simulink subsystem "Baseline"  (R2024a)
settings: Solver=VariableStepAuto  StartTime=0.0  StopTime=10.0  RelTol=1e-3
undefined symbols (not defined in the file): Baseline, ControllersLib, SimIn, SimPar
libraries: ComponentsLib x12, AdaptiveLib x1, libAxisTransformations x1
settings Model: Creator=tbritton  LastModifiedBy=azmol
settings SolverCC: AlgebraicLoopSolver=TrustRegion
settings OptimizationCC: ReuseModelBlockBuffer=off
settings DebuggingCC: UnconnectedInputMsg=warning  UnconnectedOutputMsg=warning  UnconnectedLineMsg=warning
settings ModelReferenceCC: EnableRefExpFcnMdlSchedulingChecks=on
settings RTWCC: GPUComputeCapability=3.5  DLArmComputeVersion=19.05

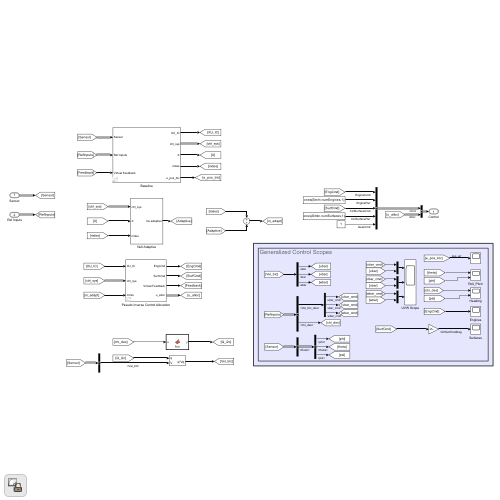
[thumbnail: Simulink's stored preview of the top-level diagram]
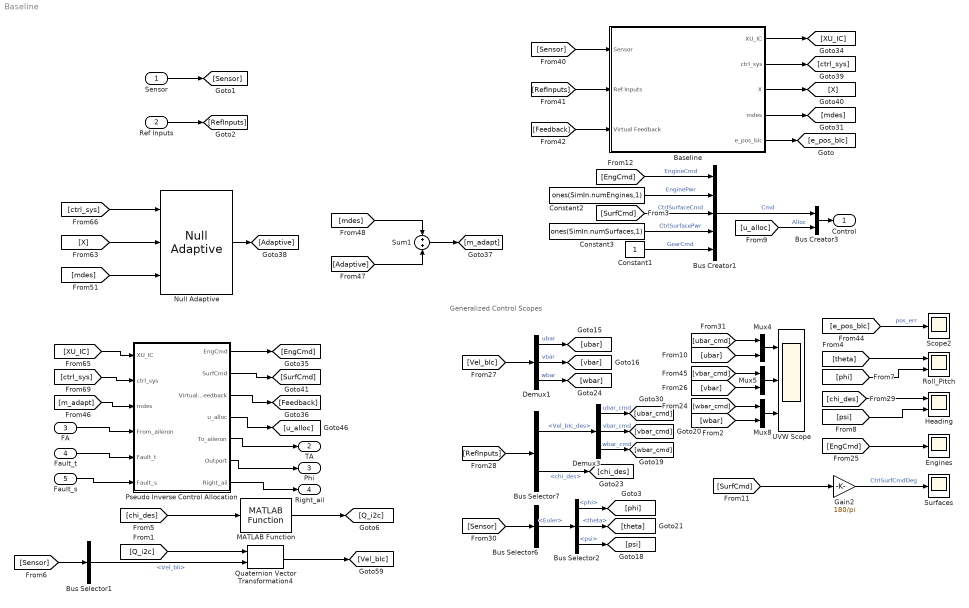
== system Baseline ==
  note: Generalized Control Scopes
  Sensor : Inport  OutDataTypeStr=Bus: SensorBus
  Ref Inputs : Inport  Port=2  OutDataTypeStr=Bus: BUS_REF_INPUT
  FA : Inport  Port=3
  Fault_t : Inport  Port=4
  Fault_s : Inport  Port=5
  Baseline : Subsystem  AncestorBlock=ControllersLib/Baseline
      settings: LibrarySourceBlock=ControllersLib/Baseline
  Bus Creator1 : BusCreator  Inputs=5  OutDataTypeStr=Bus: BUS_CMD
  Bus Creator3 : BusCreator  Inputs=2
  Bus Selector1 : BusSelector  OutputSignals=Vel_bIi
  Bus Selector2 : BusSelector  OutputSignals=phi,theta,psi
  Bus Selector6 : BusSelector  OutputSignals=Euler
  Bus Selector7 : BusSelector  OutputSignals=Vel_bIc_des,chi_des
  Constant1 : Constant
  Constant2 : Constant  Value=ones(SimIn.numEngines,1)
  Constant3 : Constant  Value=ones(SimIn.numSurfaces,1)
  Demux1 : Demux  Outputs=3
  Demux3 : Demux  Outputs=3
  Engines : Scope
  Gain2 : Gain  Gain=180/pi
  Heading : Scope  NumInputPorts=2
  MATLAB Function : ComponentsLib/ConvertToControlFrame/MATLAB Function  SystemSampleTime=-1  VariantActivationTime=update diagram  AllowFlexibleInterface=on  Latency=0  AutoFrameSizeCalculation=off
      settings: SourceProductName=Components
  Mux4 : Mux  Inputs=2
  Mux5 : Mux  Inputs=2
  Mux8 : Mux  Inputs=2
  Null Adaptive : AdaptiveLib/Null Adaptive  SystemSampleTime=-1  VariantActivationTime=update diagram  AllowFlexibleInterface=on  Latency=0  AutoFrameSizeCalculation=off
      settings: SourceProductName=Adaptive Augmentation
  Pseudo Inverse Control Allocation : Subsystem  AncestorBlock=AllocatorsLib/Pseudo Inverse Control Allocation
      settings: LibrarySourceBlock=AllocatorsLib/Pseudo Inverse Control Allocation
  Quaternion Vector Transformation4 : libAxisTransformations/Quaternion Vector Transformation  n=0
  Roll_Pitch : Scope  NumInputPorts=2
  Scope2 : Scope
  Sum1 : Sum
  Surfaces : Scope
  UVW Scope : Scope  NumInputPorts=3
  Control : Outport  OutDataTypeStr=Bus: BUS_CONTROL  VectorParamsAs1DForOutWhenUnconnected=off
  TA : Outport  Port=2
  Phi : Outport  Port=3
  Right_ail : Outport  Port=4
  wires:
  Baseline/5(e_pos_blc) -> [e_pos_bIc]
  Demux1/1 -> [ubar]  "ubar"
  Mux4/1 -> UVW Scope/1
  Demux3/3 -> [wbar_cmd]  "wbar_cmd"
  Mux5/1 -> UVW Scope/2
  [vbar_cmd] -> Mux5/1
  [ubar_cmd] -> Mux4/1
  [vbar] -> Mux5/2
  [SurfCmd] -> Gain2/1
  [chi_des] -> Heading/1
  [ubar] -> Mux4/2
  [Sensor] -> Bus Selector6/1
  [RefInputs] -> Bus Selector7/1
  [wbar] -> Mux8/2
  [phi] -> Roll_Pitch/2
  Demux3/2 -> [vbar_cmd]  "vbar_cmd"
  [e_pos_bIc] -> Scope2/1  "pos_err"
  Bus Selector6/1 -> Bus Selector2/1  "<Euler>"
  Bus Selector2/1 -> [phi]  "<phi>"
  Mux8/1 -> UVW Scope/3
  Bus Selector2/3 -> [psi]  "<psi>"
  Gain2/1 -> Surfaces/1  "CtrlSurfCmdDeg"
  [theta] -> Roll_Pitch/1
  Bus Selector2/2 -> [theta]  "<theta>"
  [psi] -> Heading/2
  Demux1/2 -> [vbar]  "vbar"
  [EngCmd] -> Engines/1
  Bus Selector7/1 -> Demux3/1  "<Vel_bIc_des>"
  Demux3/1 -> [ubar_cmd]  "ubar_cmd"
  [Vel_bIc] -> Demux1/1
  Bus Selector7/2 -> [chi_des]  "<chi_des>"
  [wbar_cmd] -> Mux8/1
  Demux1/3 -> [wbar]  "wbar"
  [Sensor] -> Bus Selector1/1
  MATLAB Function/1 -> [Q_i2c]
  Quaternion Vector Transformation4/1 -> [Vel_bIc]
  [chi_des] -> MATLAB Function/1
  [Q_i2c] -> Quaternion Vector Transformation4/1
  Bus Selector1/1 -> Quaternion Vector Transformation4/2  "<Vel_bIi>"
  [ctrl_sys] -> Pseudo Inverse Control Allocation/2(ctrl_sys)
  [XU_IC] -> Pseudo Inverse Control Allocation/1(XU_IC)
  Pseudo Inverse Control Allocation/4(u_alloc) -> [u_alloc]
  Pseudo Inverse Control Allocation/2(SurfCmd) -> [SurfCmd]
  [Adaptive] -> Sum1/2
  [mdes] -> Sum1/1
  Sum1/1 -> [m_adapt]
  Baseline/3(X) -> [X]
  Baseline/2(ctrl_sys) -> [ctrl_sys]
  Null Adaptive/1 -> [Adaptive]
  [X] -> Null Adaptive/2
  [mdes] -> Null Adaptive/3
  [ctrl_sys] -> Null Adaptive/1
  Pseudo Inverse Control Allocation/1(EngCmd) -> [EngCmd]
  Baseline/1(XU_IC) -> [XU_IC]
  Pseudo Inverse Control Allocation/3(Virtual Feedback) -> [Feedback]
  [m_adapt] -> Pseudo Inverse Control Allocation/3(mdes)
  Baseline/4(mdes) -> [mdes]
  [Feedback] -> Baseline/3(Virtual Feedback)
  [RefInputs] -> Baseline/2(Ref Inputs)
  [Sensor] -> Baseline/1(Sensor)
  Constant3/1 -> Bus Creator1/4  "CtrlSurfacePwr"
  Constant2/1 -> Bus Creator1/2  "EnginePwr"
  [EngCmd] -> Bus Creator1/1  "EngineCmd"
  Sensor/1 -> [Sensor]
  Bus Creator1/1 -> Bus Creator3/1  "Cmd"
  [SurfCmd] -> Bus Creator1/3  "CtrlSurfaceCmd"
  Constant1/1 -> Bus Creator1/5  "GearCmd"
  Bus Creator3/1 -> Control/1
  [u_alloc] -> Bus Creator3/2  "Alloc"
  Ref Inputs/1 -> [RefInputs]
  FA/1 -> Pseudo Inverse Control Allocation/4(From_aileron)
  Pseudo Inverse Control Allocation/5(To_aileron) -> TA/1
  Pseudo Inverse Control Allocation/6(Outport) -> Phi/1
  Fault_t/1 -> Pseudo Inverse Control Allocation/5(Fault_t)
  Fault_s/1 -> Pseudo Inverse Control Allocation/6(Fault_s)
  Pseudo Inverse Control Allocation/7(Right_ail) -> Right_ail/1

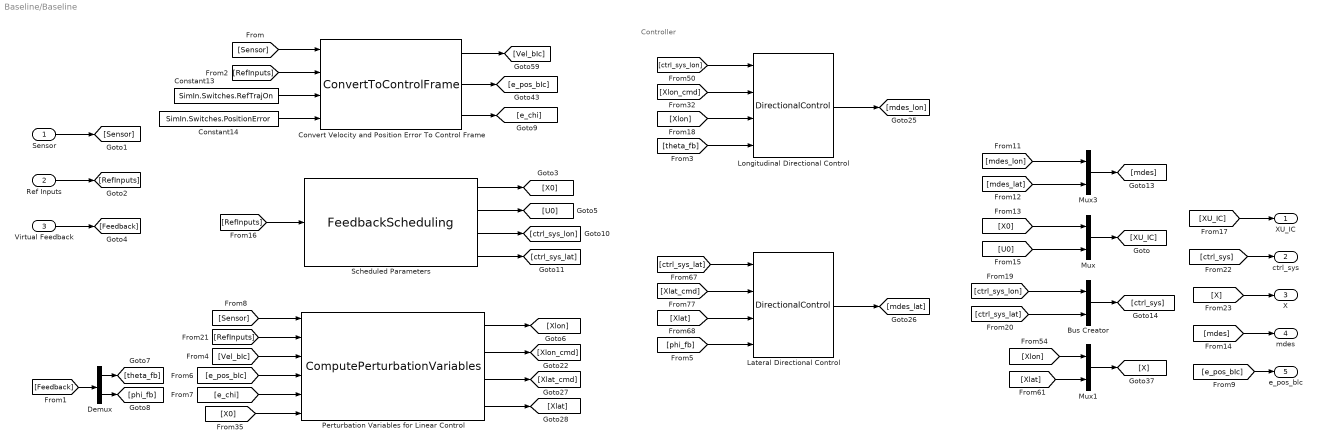
== system Baseline/Baseline ==
  note: Controller
  Sensor : Inport  OutDataTypeStr=Bus: SensorBus
  Ref Inputs : Inport  Port=2  OutDataTypeStr=Bus: BUS_REF_INPUT
  Virtual Feedback : Inport  Port=3
  Bus Creator : BusCreator  Inputs=2
  Constant13 : Constant  Value=SimIn.Switches.RefTrajOn
  Constant14 : Constant  Value=SimIn.Switches.PositionError
  Convert Velocity and Position Error To Control Frame : ComponentsLib/ConvertToControlFrame  SystemSampleTime=-1  VariantActivationTime=update diagram  AllowFlexibleInterface=on  Latency=0  AutoFrameSizeCalculation=off
      settings: SourceProductName=Components
  Demux : Demux  Outputs=2
  Lateral Directional Control : ComponentsLib/DirectionalControl  SystemSampleTime=-1  VariantActivationTime=update diagram  AllowFlexibleInterface=on  Latency=0  AutoFrameSizeCalculation=off
      settings: SourceProductName=Components
  Longitudinal Directional Control : ComponentsLib/DirectionalControl  SystemSampleTime=-1  VariantActivationTime=update diagram  AllowFlexibleInterface=on  Latency=0  AutoFrameSizeCalculation=off
      settings: SourceProductName=Components
  Mux : Mux  Inputs=2
  Mux1 : Mux  Inputs=2
  Mux3 : Mux  Inputs=2
  Perturbation Variables for Linear Control : ComponentsLib/ComputePerturbationVariables  SystemSampleTime=-1  VariantActivationTime=update diagram  AllowFlexibleInterface=on  Latency=0  AutoFrameSizeCalculation=off
      settings: SourceProductName=Components
  Scheduled Parameters : ComponentsLib/FeedbackScheduling  SystemSampleTime=-1  VariantActivationTime=update diagram  AllowFlexibleInterface=on  Latency=0  AutoFrameSizeCalculation=off
      settings: SourceProductName=Components
  XU_IC : Outport
  ctrl_sys : Outport  Port=2
  X : Outport  Port=3
  mdes : Outport  Port=4
  e_pos_blc : Outport  Port=5
  wires:
  [X] -> X/1
  [Xlat] -> Mux1/2
  [Xlon] -> Mux1/1
  Mux1/1 -> [X]
  [ctrl_sys] -> ctrl_sys/1
  Bus Creator/1 -> [ctrl_sys]
  [ctrl_sys_lat] -> Bus Creator/2
  [ctrl_sys_lon] -> Bus Creator/1
  [XU_IC] -> XU_IC/1
  Mux/1 -> [XU_IC]
  [U0] -> Mux/2
  [X0] -> Mux/1
  [mdes] -> mdes/1
  Mux3/1 -> [mdes]
  [mdes_lat] -> Mux3/2
  [mdes_lon] -> Mux3/1
  [phi_fb] -> Lateral Directional Control/4
  [theta_fb] -> Longitudinal Directional Control/4
  Demux/1 -> [theta_fb]
  Demux/2 -> [phi_fb]
  [Feedback] -> Demux/1
  Virtual Feedback/1 -> [Feedback]
  [Xlat_cmd] -> Lateral Directional Control/2
  [Xlon] -> Longitudinal Directional Control/3
  [Xlat] -> Lateral Directional Control/3
  Longitudinal Directional Control/1 -> [mdes_lon]
  [ctrl_sys_lon] -> Longitudinal Directional Control/1
  [ctrl_sys_lat] -> Lateral Directional Control/1
  Lateral Directional Control/1 -> [mdes_lat]
  [Xlon_cmd] -> Longitudinal Directional Control/2
  Scheduled Parameters/4 -> [ctrl_sys_lat]
  Scheduled Parameters/2 -> [U0]
  [e_chi] -> Perturbation Variables for Linear Control/5
  Constant14/1 -> Convert Velocity and Position Error To Control Frame/4
  [RefInputs] -> Perturbation Variables for Linear Control/2
  Constant13/1 -> Convert Velocity and Position Error To Control Frame/3
  [Vel_bIc] -> Perturbation Variables for Linear Control/3
  [Sensor] -> Convert Velocity and Position Error To Control Frame/1
  Convert Velocity and Position Error To Control Frame/3 -> [e_chi]
  Perturbation Variables for Linear Control/2 -> [Xlon_cmd]
  [RefInputs] -> Scheduled Parameters/1
  Perturbation Variables for Linear Control/4 -> [Xlat]
  [e_pos_bIc] -> Perturbation Variables for Linear Control/4
  Scheduled Parameters/3 -> [ctrl_sys_lon]
  Convert Velocity and Position Error To Control Frame/2 -> [e_pos_bIc]
  Convert Velocity and Position Error To Control Frame/1 -> [Vel_bIc]
  [RefInputs] -> Convert Velocity and Position Error To Control Frame/2
  Ref Inputs/1 -> [RefInputs]
  Scheduled Parameters/1 -> [X0]
  Sensor/1 -> [Sensor]
  Perturbation Variables for Linear Control/3 -> [Xlat_cmd]
  [Sensor] -> Perturbation Variables for Linear Control/1
  Perturbation Variables for Linear Control/1 -> [Xlon]
  [X0] -> Perturbation Variables for Linear Control/6
  [e_pos_bIc] -> e_pos_blc/1

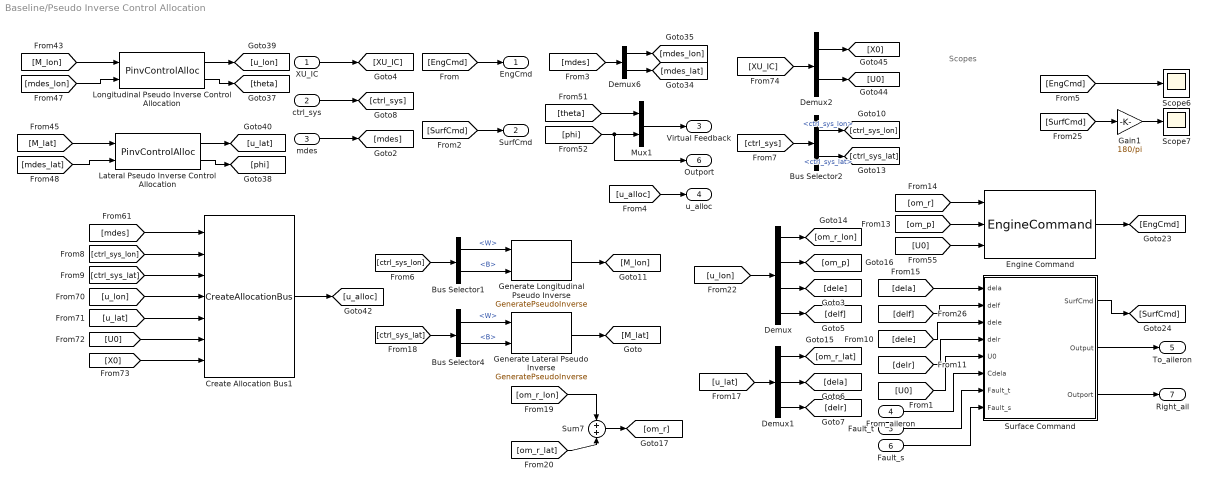
== system Baseline/Pseudo Inverse Control Allocation ==
  note: Scopes
  XU_IC : Inport
  ctrl_sys : Inport  Port=2
  mdes : Inport  Port=3
  From_aileron : Inport  Port=4
  Fault_t : Inport  Port=5
  Fault_s : Inport  Port=6
  Bus Selector1 : BusSelector  OutputSignals=W,B
  Bus Selector2 : BusSelector  OutputSignals=ctrl_sys_lon,ctrl_sys_lat
  Bus Selector4 : BusSelector  OutputSignals=W,B
  Create Allocation Bus1 : ComponentsLib/CreateAllocationBus  SystemSampleTime=-1  VariantActivationTime=update diagram  AllowFlexibleInterface=on  Latency=0  AutoFrameSizeCalculation=off
      settings: SourceProductName=Components
  Demux : Demux  Outputs=[8 1 1 1]
  Demux1 : Demux  Outputs=[8 1 1]
  Demux2 : Demux  Outputs=[12 13]
  Demux6 : Demux  Outputs=[3 3]
  Engine Command : ComponentsLib/EngineCommand  SystemSampleTime=-1  VariantActivationTime=update diagram  AllowFlexibleInterface=on  Latency=0  AutoFrameSizeCalculation=off
      settings: SourceProductName=Components
  Gain1 : Gain  Gain=180/pi
  Generate Lateral Pseudo Inverse : ComponentsLib/GeneratePseudoInverse  SystemSampleTime=-1  VariantActivationTime=update diagram  AllowFlexibleInterface=on  Latency=0  AutoFrameSizeCalculation=off
      settings: SourceProductName=Components
  Generate Longitudinal Pseudo Inverse : ComponentsLib/GeneratePseudoInverse  SystemSampleTime=-1  VariantActivationTime=update diagram  AllowFlexibleInterface=on  Latency=0  AutoFrameSizeCalculation=off
      settings: SourceProductName=Components
  Lateral Pseudo Inverse Control Allocation : ComponentsLib/PinvControlAlloc  SystemSampleTime=-1  VariantActivationTime=update diagram  AllowFlexibleInterface=on  Latency=0  AutoFrameSizeCalculation=off
      settings: SourceProductName=Components
  Longitudinal Pseudo Inverse Control Allocation : ComponentsLib/PinvControlAlloc  SystemSampleTime=-1  VariantActivationTime=update diagram  AllowFlexibleInterface=on  Latency=0  AutoFrameSizeCalculation=off
      settings: SourceProductName=Components
  Mux1 : Mux  Inputs=2
  Scope6 : Scope
  Scope7 : Scope
  Sum7 : Sum
  Surface Command : Subsystem  AncestorBlock=ComponentsLib/SurfaceCommand
  EngCmd : Outport
  SurfCmd : Outport  Port=2
  Virtual Feedback : Outport  Port=3
  u_alloc : Outport  Port=4
  To_aileron : Outport  Port=5
  Outport : Outport  Port=6
  Right_ail : Outport  Port=7
  wires:
  Surface Command/3(Outport) -> Right_ail/1
  Fault_s/1 -> Surface Command/8(Fault_s)
  Fault_t/1 -> Surface Command/7(Fault_t)
  From_aileron/1 -> Surface Command/6(Cdela)
  Surface Command/2(Output) -> To_aileron/1
  [ctrl_sys_lat] -> Create Allocation Bus1/3
  [ctrl_sys_lon] -> Create Allocation Bus1/2
  Bus Selector2/2 -> [ctrl_sys_lat]  "<ctrl_sys_lat>"
  Bus Selector2/1 -> [ctrl_sys_lon]  "<ctrl_sys_lon>"
  [ctrl_sys] -> Bus Selector2/1
  Bus Selector1/2 -> Generate Longitudinal Pseudo Inverse/2  "<B>"
  Bus Selector4/2 -> Generate Lateral Pseudo Inverse/2  "<B>"
  Generate Lateral Pseudo Inverse/1 -> [M_lat]
  Bus Selector4/1 -> Generate Lateral Pseudo Inverse/1  "<W>"
  Generate Longitudinal Pseudo Inverse/1 -> [M_lon]
  [ctrl_sys_lon] -> Bus Selector1/1
  Bus Selector1/1 -> Generate Longitudinal Pseudo Inverse/1  "<W>"
  [ctrl_sys_lat] -> Bus Selector4/1
  [EngCmd] -> Scope6/1
  [SurfCmd] -> Gain1/1
  Gain1/1 -> Scope7/1
  [u_alloc] -> u_alloc/1
  ctrl_sys/1 -> [ctrl_sys]
  XU_IC/1 -> [XU_IC]
  mdes/1 -> [mdes]
  [mdes] -> Demux6/1
  Demux6/1 -> [mdes_lon]
  Demux6/2 -> [mdes_lat]
  [mdes] -> Create Allocation Bus1/1
  Demux2/1 -> [X0]
  [X0] -> Create Allocation Bus1/7
  [XU_IC] -> Demux2/1
  [u_lat] -> Create Allocation Bus1/5
  Create Allocation Bus1/1 -> [u_alloc]
  [u_lon] -> Create Allocation Bus1/4
  [U0] -> Create Allocation Bus1/6
  Demux2/2 -> [U0]
  [SurfCmd] -> SurfCmd/1
  [EngCmd] -> EngCmd/1
  [dela] -> Surface Command/1(dela)
  [U0] -> Surface Command/5(U0)
  [om_r] -> Engine Command/1
  [om_p] -> Engine Command/2
  [delr] -> Surface Command/4(delr)
  [delf] -> Surface Command/2(delf)
  [dele] -> Surface Command/3(dele)
  [U0] -> Engine Command/3
  Surface Command/1(SurfCmd) -> [SurfCmd]
  Engine Command/1 -> [EngCmd]
  Demux1/3 -> [delr]
  Demux/4 -> [delf]
  Demux/1 -> [om_r_lon]
  Demux1/1 -> [om_r_lat]
  Demux1/2 -> [dela]
  [u_lon] -> Demux/1
  Sum7/1 -> [om_r]
  [om_r_lon] -> Sum7/1
  [om_r_lat] -> Sum7/2
  [u_lat] -> Demux1/1
  Demux/2 -> [om_p]
  Demux/3 -> [dele]
  [M_lat] -> Lateral Pseudo Inverse Control Allocation/1
  [M_lon] -> Longitudinal Pseudo Inverse Control Allocation/1
  Mux1/1 -> Virtual Feedback/1
  Longitudinal Pseudo Inverse Control Allocation/2 -> [theta]
  Lateral Pseudo Inverse Control Allocation/1 -> [u_lat]
  [mdes_lon] -> Longitudinal Pseudo Inverse Control Allocation/2
  [phi] -> Mux1/2, Outport/1
  [mdes_lat] -> Lateral Pseudo Inverse Control Allocation/2
  [theta] -> Mux1/1
  Longitudinal Pseudo Inverse Control Allocation/1 -> [u_lon]
  Lateral Pseudo Inverse Control Allocation/2 -> [phi]

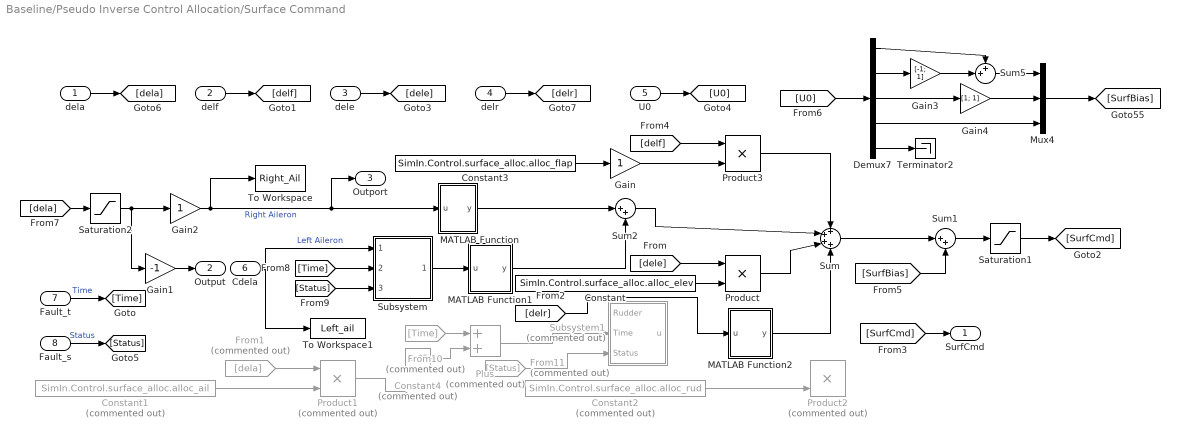
== system Baseline/Pseudo Inverse Control Allocation/Surface Command ==
  dela : Inport
  delf : Inport  Port=2
  dele : Inport  Port=3
  delr : Inport  Port=4
  U0 : Inport  Port=5
  Cdela : Inport  Port=6
  Fault_t : Inport  Port=7
  Fault_s : Inport  Port=8
  Constant : Constant  Value=SimIn.Control.surface_alloc.alloc_elev
  Constant1 : Constant  Commented=on  Value=SimIn.Control.surface_alloc.alloc_ail
  Constant2 : Constant  Commented=on  Value=SimIn.Control.surface_alloc.alloc_rud
  Constant3 : Constant  Value=SimIn.Control.surface_alloc.alloc_flap
  Constant4 : Constant  Commented=on  Value=-0.05
  Demux7 : Demux  Outputs=[1 1 1 1 -1]
  From1 : From  Commented=on  GotoTag=dela
  From10 : From  Commented=on  GotoTag=Time
  From11 : From  Commented=on  GotoTag=Status
  Gain : Gain
  Gain1 : Gain  Gain=-1
  Gain2 : Gain
  Gain3 : Gain  Gain=[-1; 1]
  Gain4 : Gain  Gain=[1; 1]
  MATLAB Function : MATLAB Function  TreatAsAtomicUnit=on
  MATLAB Function1 : MATLAB Function  TreatAsAtomicUnit=on
  MATLAB Function2 : MATLAB Function  TreatAsAtomicUnit=on
  Mux4 : Mux  Inputs=3
  Plus : Sum  Commented=on
  Product : Product
  Product1 : Product  Commented=on
  Product2 : Product  Commented=on
  Product3 : Product
  Saturation1 : Saturate  UpperLimit=SimPar.Actuator.MaxPos  LowerLimit=SimPar.Actuator.MinPos
  Saturation2 : Saturate  UpperLimit=0.44  LowerLimit=-0.44
  Subsystem : Subsystem
  Subsystem1 : Subsystem  Commented=on
  Sum : Sum  Inputs=++++
  Sum1 : Sum  Inputs=|++
  Sum2 : Sum  Inputs=|++
  Sum5 : Sum  Inputs=++|
  Terminator2 : Terminator
  To Workspace : ToWorkspace  VariableName=Right_Ail  SaveFormat=Timeseries  SampleTime=-1
  To Workspace1 : ToWorkspace  VariableName=Left_ail  SaveFormat=Timeseries  SampleTime=-1
  SurfCmd : Outport
  Output : Outport  Port=2
  Outport : Outport  Port=3
  wires:
  [delr] -> MATLAB Function2/1(u)
  From11/1 -> Subsystem1/3(Status)
  Plus/1 -> Subsystem1/2(Time)
  [Status] -> Subsystem/3(Inport1)
  [Time] -> Subsystem/2(Inport)
  Fault_s/1 -> [Status]  "Status"
  Fault_t/1 -> [Time]  "Time"
  Constant2/1 -> Product2/2
  Subsystem/1(Out1) -> MATLAB Function1/1(u)
  Cdela/1 -> Subsystem/1(Left Aileron), To Workspace1/1  "Left Aileron"
  Saturation2/1 -> Gain1/1, Gain2/1
  MATLAB Function1/1(y) -> Sum2/2
  MATLAB Function/1(y) -> Sum2/1
  Gain1/1 -> Output/1
  Gain2/1 -> To Workspace/1, MATLAB Function/1(u), Outport/1  "Right Aileron"
  [dela] -> Saturation2/1
  Gain/1 -> Product3/2
  [delf] -> Product3/1
  Constant3/1 -> Gain/1
  Product3/1 -> Sum/1
  [SurfBias] -> Sum1/2
  Sum/1 -> Sum1/1
  Sum1/1 -> Saturation1/1
  MATLAB Function2/1(y) -> Sum/4
  Product/1 -> Sum/3
  Constant/1 -> Product/2
  [dele] -> Product/1
  U0/1 -> [U0]
  Gain4/1 -> Mux4/2
  Demux7/1 -> Sum5/1
  Demux7/5 -> Terminator2/1
  Gain3/1 -> Sum5/2
  Demux7/3 -> Gain4/1
  Demux7/4 -> Mux4/3
  [U0] -> Demux7/1
  Mux4/1 -> [SurfBias]
  Demux7/2 -> Gain3/1
  Sum5/1 -> Mux4/1
  Saturation1/1 -> [SurfCmd]
  [SurfCmd] -> SurfCmd/1
  delf/1 -> [delf]
  delr/1 -> [delr]
  dela/1 -> [dela]
  dele/1 -> [dele]
  From1/1 -> Product1/1
  Constant1/1 -> Product1/2
  Product1/1 -> ?
  Sum2/1 -> Sum/2
  From10/1 -> Plus/1
  Constant4/1 -> Plus/2

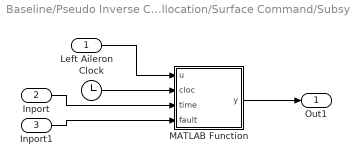
== system Baseline/Pseudo Inverse Control Allocation/Surface Command/Subsystem ==
  Left Aileron : Inport
  Inport : Inport  Port=2
  Inport1 : Inport  Port=3
  Clock : Clock
  MATLAB Function : MATLAB Function  TreatAsAtomicUnit=on
  Out1 : Outport
  wires:
  Inport1/1 -> MATLAB Function/4(fault)
  Inport/1 -> MATLAB Function/3(time)
  MATLAB Function/1(y) -> Out1/1
  Left Aileron/1 -> MATLAB Function/1(u)
  Clock/1 -> MATLAB Function/2(cloc)

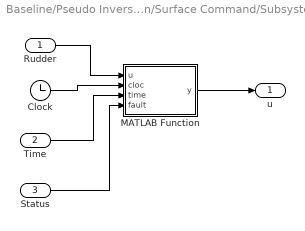
== system Baseline/Pseudo Inverse Control Allocation/Surface Command/Subsystem1 ==
  Rudder : Inport
  Time : Inport  Port=2
  Status : Inport  Port=3
  Clock : Clock
  MATLAB Function : MATLAB Function  TreatAsAtomicUnit=on
  u : Outport
  wires:
  MATLAB Function/1(y) -> u/1
  Rudder/1 -> MATLAB Function/1(u)
  Clock/1 -> MATLAB Function/2(cloc)
  Time/1 -> MATLAB Function/3(time)
  Status/1 -> MATLAB Function/4(fault)

== matlab function Baseline/Pseudo Inverse Control Allocation/Surface Command/MATLAB Function ==
  data: u input; y output
function y = fcn(u)

k = [0;1;0;0;0];
y = u.*k;

== matlab function Baseline/Pseudo Inverse Control Allocation/Surface Command/MATLAB Function1 ==
  data: u input; y output
function y = fcn(u)

k = [1;0;0;0;0];
y = u.*k;

== matlab function Baseline/Pseudo Inverse Control Allocation/Surface Command/Subsystem/MATLAB Function ==
  data: u input; y output; cloc input; time input; fault input
function y = fcn(u, cloc, time, fault)

y = u;

if cloc >= time && fault == 1
    %y = u.*0.3;
    y = u+0.08;
end

== matlab function Baseline/Pseudo Inverse Control Allocation/Surface Command/MATLAB Function2 ==
  data: u input; y output
function y = fcn(u)

k = [0;0;0;0;1];
y = u.*k;

== matlab function Baseline/Pseudo Inverse Control Allocation/Surface Command/Subsystem1/MATLAB Function ==
  data: u input; y output; cloc input; time input; fault input
function y = fcn(u, cloc, time, fault)

y = u;

if cloc >= time && fault == 1
    %y = u.*0.3;
    y = u-0.3;
end
